simulink model "BulbaBot_ControlLoop"  (R2021b)
settings: Solver=FixedStepAuto  StartTime=0.0  StopTime=2  FixedStep=1e-5  RelTol=1e-3
model workspace (MAT data in the model file):
  PWM_sampleTime = 1e-05
  xG = 0.01
  xd = 189
  yG = 0.01
  yd = 130
  zG = 0.01
  zd = -23
undefined symbols (not defined in the file or in its folder): DiscIntNeverNeededParam
libraries: spsMeanLib x3, simulink x3
settings Model: Creator=Alessandro  LastModifiedBy=Alessandro
settings DataIOCC: ReturnWorkspaceOutputs=off

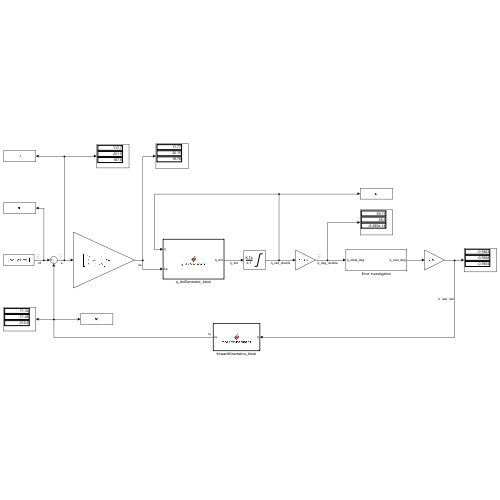
[thumbnail: Simulink's stored preview of the top-level diagram]
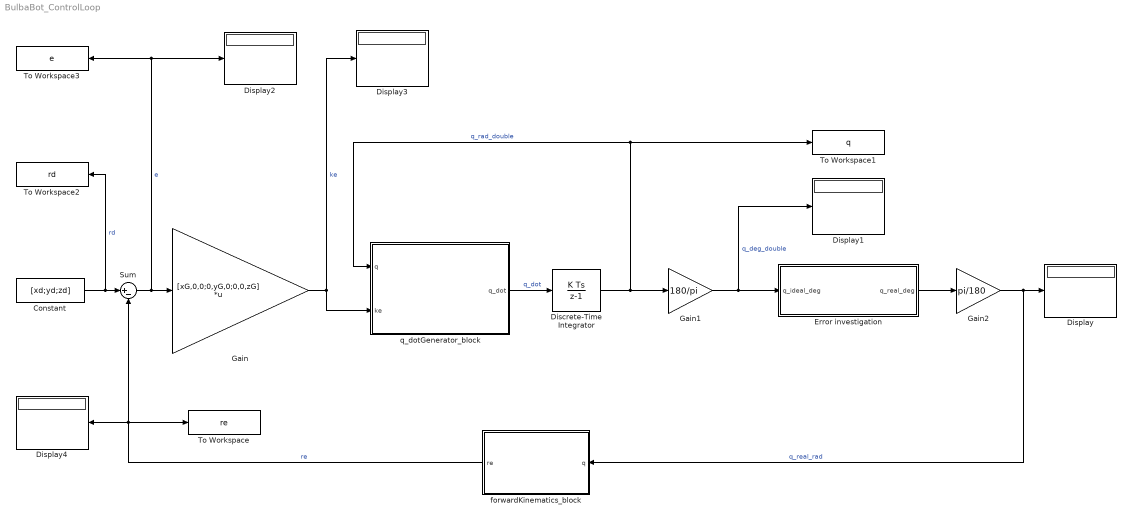
== system BulbaBot_ControlLoop ==
  Constant : Constant  Value=[xd;yd;zd]
  Discrete-Time Integrator : DiscreteIntegrator  InitialCondition=[0,0,0]  SampleTime=-1  LimitOutput=on  UpperSaturationLimit=[pi,pi,pi]  LowerSaturationLimit=[-pi,-pi,-pi]  ICPrevOutput=DiscIntNeverNeededParam  ICPrevScaledInput=DiscIntNeverNeededParam
  Display{,1..4} (5 alike) : Display
  Error investigation : Subsystem
  Gain : Gain  Gain=[xG,0,0;0,yG,0;0,0,zG]  Multiplication=Matrix(K*u)
  Gain1 : Gain  Gain=180/pi
  Gain2 : Gain  Gain=pi/180
  Sum : Sum  Inputs=|+-
  To Workspace : ToWorkspace  VariableName=re  SaveFormat=Timeseries  SampleTime=-1
  To Workspace1 : ToWorkspace  VariableName=q  SaveFormat=Timeseries  SampleTime=-1
  To Workspace2 : ToWorkspace  VariableName=rd  SaveFormat=Timeseries  SampleTime=-1
  To Workspace3 : ToWorkspace  VariableName=e  SaveFormat=Timeseries  SampleTime=-1
  forwardKinematics_block : MATLAB Function  TreatAsAtomicUnit=on
  q_dotGenerator_block : MATLAB Function  TreatAsAtomicUnit=on
  wires:
  Constant/1 -> To Workspace2/1, Sum/1  "rd"
  forwardKinematics_block/1(re) -> To Workspace/1, Display4/1, Sum/2  "re"
  Gain/1 -> q_dotGenerator_block/2(ke), Display3/1  "ke"
  Gain1/1 -> Error investigation/1(q_ideal_deg), Display1/1  "q_deg_double"
  Discrete-Time Integrator/1 -> To Workspace1/1, q_dotGenerator_block/1(q), Gain1/1  "q_rad_double"
  Sum/1 -> To Workspace3/1, Display2/1, Gain/1  "e"
  q_dotGenerator_block/1(q_dot) -> Discrete-Time Integrator/1  "q_dot"
  Gain2/1 -> forwardKinematics_block/1(q), Display/1  "q_real_rad"
  Error investigation/1(q_real_deg) -> Gain2/1

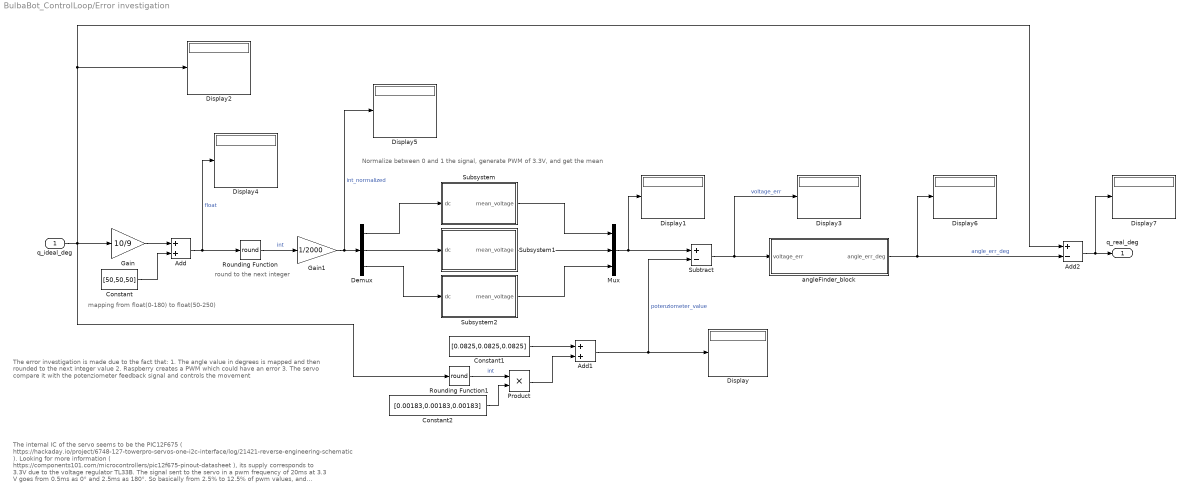
== system BulbaBot_ControlLoop/Error investigation ==
  note: Normalize between 0 and 1 the signal, generate PWM of 3.3V, and get the mean
  note: The internal IC of the servo seems to be the PIC12F675 ( https://hackaday.io/project/6748-127-towerpro-servos-one-i2c-interface/log/21421-reverse-engineering-schematic ).
      |
      | Looking for more information ( https://components101.com/microcontrollers/pic12f675-pinout-datasheet ), its supply corresponds to 3.3V due to the voltage regulator TL33B.
      |
      | The signal sent to the servo in a pwm frequency of 20ms at 3.3 V goes from 0.5ms as 0° and 2.5ms as 180°.
      | So basically from 2.5% to 12.5% of pwm values, and [0.0825,0.4125] V.
  note: round to the next integer
  note: mapping from float(0-180) to float(50-250)
  note: The error investigation is made due to the fact that:
      |
      | 1. The angle value in degrees is mapped and then rounded to the next integer value
      | 2. Raspberry creates a PWM which could have an error
      | 3. The servo compare it with the potenziometer feedback signal and controls the movement
  q_ideal_deg : Inport
  Add : Sum
  Add1 : Sum
  Add2 : Sum  Inputs=+-
  Constant : Constant  Value=[50,50,50]
  Constant1 : Constant  Value=[0.0825,0.0825,0.0825]
  Constant2 : Constant  Value=[0.00183,0.00183,0.00183]
  Demux : Demux  Outputs=3
  Display{,1..7} (8 alike) : Display
  Gain : Gain  Gain=10/9
  Gain1 : Gain  Gain=1/2000
  Mux : Mux  Inputs=3
  Product : Product
  Rounding Function : Rounding  Operator=round
  Rounding Function1 : Rounding  Operator=round
  Subsystem : Subsystem
  Subsystem1 : Subsystem
  Subsystem2 : Subsystem
  Subtract : Sum  Inputs=+-
  angleFinder_block : MATLAB Function  TreatAsAtomicUnit=on
  q_real_deg : Outport
  wires:
  q_ideal_deg/1 -> Add2/1, Display2/1, Rounding Function1/1, Gain/1
  Gain/1 -> Add/1
  Add/1 -> Rounding Function/1, Display4/1  "float"
  Constant/1 -> Add/2
  Rounding Function/1 -> Gain1/1  "int"
  Subtract/1 -> Display3/1, angleFinder_block/1(voltage_err)  "voltage_err"
  angleFinder_block/1(angle_err_deg) -> Add2/2, Display6/1  "angle_err_deg"
  Mux/1 -> Subtract/1, Display1/1
  Gain1/1 -> Display5/1, Demux/1  "int_normalized"
  Demux/1 -> Subsystem/1(dc)
  Demux/2 -> Subsystem1/1(dc)
  Demux/3 -> Subsystem2/1(dc)
  Subsystem/1(mean_voltage) -> Mux/1
  Subsystem1/1(mean_voltage) -> Mux/2
  Subsystem2/1(mean_voltage) -> Mux/3
  Add1/1 -> Subtract/2, Display/1  "potenziometer_value"
  Constant1/1 -> Add1/1
  Product/1 -> Add1/2
  Rounding Function1/1 -> Product/1  "int"
  Constant2/1 -> Product/2
  Add2/1 -> Display7/1, q_real_deg/1

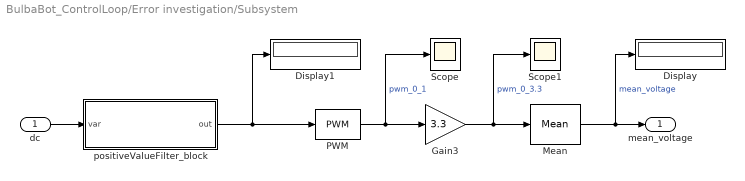
== system BulbaBot_ControlLoop/Error investigation/Subsystem ==
  dc : Inport
  Display : Display
  Display1 : Display
  Gain3 : Gain  Gain=3.3
  Mean : spsMeanLib/Mean  Freq=50  Vinit=0  Ts=0
  PWM : simulink/Discontinuities/PWM  DisableCoverage=on  Period=0.02  DisallowZeroDutyCycle=off  RunAtFixedTimeIntervals=on  SampleTime=PWM_sampleTime
  Scope : Scope
  Scope1 : Scope
  positiveValueFilter_block : MATLAB Function  TreatAsAtomicUnit=on
  mean_voltage : Outport
  wires:
  Gain3/1 -> Scope1/1, Mean/1  "pwm_0_3.3"
  PWM/1 -> Gain3/1, Scope/1  "pwm_0_1"
  Mean/1 -> Display/1, mean_voltage/1  "mean_voltage"
  dc/1 -> positiveValueFilter_block/1(var)
  positiveValueFilter_block/1(out) -> Display1/1, PWM/1

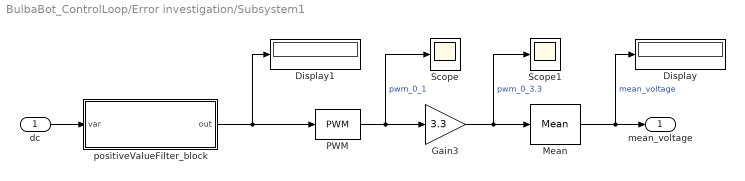
== system BulbaBot_ControlLoop/Error investigation/Subsystem1 ==
  dc : Inport
  Display : Display
  Display1 : Display
  Gain3 : Gain  Gain=3.3
  Mean : spsMeanLib/Mean  Freq=50  Vinit=0  Ts=0
  PWM : simulink/Discontinuities/PWM  DisableCoverage=on  Period=0.02  DisallowZeroDutyCycle=off  RunAtFixedTimeIntervals=on  SampleTime=PWM_sampleTime
  Scope : Scope
  Scope1 : Scope
  positiveValueFilter_block : MATLAB Function  TreatAsAtomicUnit=on
  mean_voltage : Outport
  wires:
  Gain3/1 -> Scope1/1, Mean/1  "pwm_0_3.3"
  PWM/1 -> Gain3/1, Scope/1  "pwm_0_1"
  Mean/1 -> Display/1, mean_voltage/1  "mean_voltage"
  dc/1 -> positiveValueFilter_block/1(var)
  positiveValueFilter_block/1(out) -> Display1/1, PWM/1

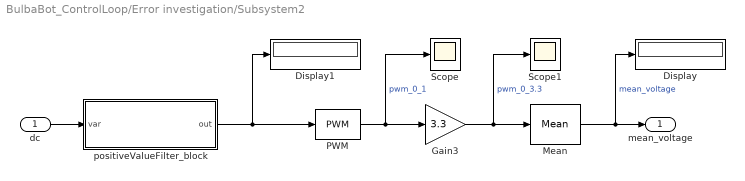
== system BulbaBot_ControlLoop/Error investigation/Subsystem2 ==
  dc : Inport
  Display : Display
  Display1 : Display
  Gain3 : Gain  Gain=3.3
  Mean : spsMeanLib/Mean  Freq=50  Vinit=0  Ts=0
  PWM : simulink/Discontinuities/PWM  DisableCoverage=on  Period=0.02  DisallowZeroDutyCycle=off  RunAtFixedTimeIntervals=on  SampleTime=PWM_sampleTime
  Scope : Scope
  Scope1 : Scope
  positiveValueFilter_block : MATLAB Function  TreatAsAtomicUnit=on
  mean_voltage : Outport
  wires:
  Gain3/1 -> Scope1/1, Mean/1  "pwm_0_3.3"
  PWM/1 -> Gain3/1, Scope/1  "pwm_0_1"
  Mean/1 -> Display/1, mean_voltage/1  "mean_voltage"
  dc/1 -> positiveValueFilter_block/1(var)
  positiveValueFilter_block/1(out) -> Display1/1, PWM/1

== matlab function BulbaBot_ControlLoop/Error investigation/Subsystem/positiveValueFilter_block ==
  data: var input; out output
function out = positiveValueFilter(var)
% DEFINITION:    Function used to delete values lower than 0

% INPUT:         var = in value

% OUTPUT:        out = only positive value or 0

    if var < 0
        out = 0;
    else
        out = var;
    end
end

== matlab function BulbaBot_ControlLoop/q_dotGenerator_block ==
  data: q input; q_dot output; ke input
function q_dot = q_dotGenerator(q,ke)
% DEFINITION:    The evaluation of the Jacobian permits to get the value of
%                q_dot, which after has been integrated begin the needed q

% INPUT:         q = quantized rounded expected angle
%                ke = results of the multiplication of the error with the gain correction

% OUTPUT:        q_dot = angular velocity in rads/s of the joints

%% Jacobian computation
%   Computation made in J_T_evaluation
    q1 = q(1);
    q2 = q(2);
    q3 = q(3);

    J1 = [- (101*sin(q1))/2 - 160*sin(q3)*((4967757600021511*cos(q1)*cos(q2))/81129638414606681695789005144064 - sin(q1)*sin(q2)) - (710389336803076073*cos(q1)*sin(q2))/162259276829213363391578010288128 - (143*cos(q2)*sin(q1))/2 - 160*cos(q3)*((4967757600021511*cos(q1)*sin(q2))/81129638414606681695789005144064 + cos(q2)*sin(q1)), - 160*sin(q3)*(cos(q1)*cos(q2) - (4967757600021511*sin(q1)*sin(q2))/81129638414606681695789005144064) - (143*cos(q1)*sin(q2))/2 - (710389336803076073*cos(q2)*sin(q1))/162259276829213363391578010288128 - 160*cos(q3)*(cos(q1)*sin(q2) + (4967757600021511*cos(q2)*sin(q1))/81129638414606681695789005144064), - 160*sin(q3)*(cos(q1)*cos(q2) - (4967757600021511*sin(q1)*sin(q2))/81129638414606681695789005144064) - 160*cos(q3)*(cos(q1)*sin(q2) + (4967757600021511*cos(q2)*sin(q1))/81129638414606681695789005144064)];
    J2 = [  (101*cos(q1))/2 - 160*sin(q3)*(cos(q1)*sin(q2) + (4967757600021511*cos(q2)*sin(q1))/81129638414606681695789005144064) + (143*cos(q1)*cos(q2))/2 - (710389336803076073*sin(q1)*sin(q2))/162259276829213363391578010288128 + 160*cos(q3)*(cos(q1)*cos(q2) - (4967757600021511*sin(q1)*sin(q2))/81129638414606681695789005144064),   (710389336803076073*cos(q1)*cos(q2))/162259276829213363391578010288128 - 160*sin(q3)*((4967757600021511*cos(q1)*sin(q2))/81129638414606681695789005144064 + cos(q2)*sin(q1)) - (143*sin(q1)*sin(q2))/2 + 160*cos(q3)*((4967757600021511*cos(q1)*cos(q2))/81129638414606681695789005144064 - sin(q1)*sin(q2)),   160*cos(q3)*((4967757600021511*cos(q1)*cos(q2))/81129638414606681695789005144064 - sin(q1)*sin(q2)) - 160*sin(q3)*((4967757600021511*cos(q1)*sin(q2))/81129638414606681695789005144064 + cos(q2)*sin(q1))];
    J3 = [                                                                                                                                                                                                                                                                                                                               0,                                                                                                                                                                                                                                                    (143*cos(q2))/2 + 160*cos(q2)*cos(q3) - 160*sin(q2)*sin(q3),                                                                                                                                                                   160*cos(q2)*cos(q3) - 160*sin(q2)*sin(q3)];
 
    J = [J1;J2;J3];

%% Result evaluation
%     q_dot = J'*ke*e
    q1_dot = J(1,1)*ke(1)+J(2,1)*ke(2)+J(3,1)*ke(3);
    q2_dot = J(1,2)*ke(1)+J(2,2)*ke(2)+J(3,2)*ke(3);
    q3_dot = J(1,3)*ke(1)+J(2,3)*ke(2)+J(3,3)*ke(3);
    q_dot = [q1_dot,q2_dot,q3_dot];
end

== matlab function BulbaBot_ControlLoop/Error investigation/angleFinder_block ==
  data: voltage_err input; angle_err_deg output
function angle_err_deg = angleFinder(voltage_err)
% DEFINITION:    Function used to map the voltage error from the
%                comparator into a real angle error that can be used to correct the
%                overral error

% INPUT:         voltage_err = output of the comparator 

% OUTPUT:        angle_err_deg = real angle error in degrees

    %map voltage error from 0/3.3 V to 0/20 ms 
    pwm_dc_err = voltage_err.*0.02./3.3;

    %map error from 0.5/2.5 ms to 0/180
    angle_err_deg = zeros(1,length(pwm_dc_err));
    for i = 1:length(pwm_dc_err)
        if abs(pwm_dc_err(i))<0.0005 %mean that the error is less than 0°
            angle_err_deg(i) = 0;
        else
            if pwm_dc_err(i) >= 0
                angle_err_deg(i) = 90000*pwm_dc_err(i)-45;
            else
                angle_err_deg(i) = pwm_dc_err(i)*90000+45;
            end
        end
    end
end

== matlab function BulbaBot_ControlLoop/forwardKinematics_block ==
  data: re output; q input
function re = forwardKinematics(q)
% DEFINITION:    after had evaluated the error of the servo through caused from
%                its internal quantization of rounded angle forward kinematics is applied
%                in order to get the expected real value of the position and use it into
%                simulink to get the error

% INPUT:         q = quantized rounded expected angle

% OUTPUT:        re = expected real position of the end effector

%% Generation of the T matrix with the aim of DH convention formula
%     With the following method the T03 matrix is evaluated at each iteration
%     T = eye(4);
%     for i = 1:3
%         T = T * [cos(q(i)),-sin(q(i))*cos(alpha(i)),sin(q(i))*sin(alpha(i)),a(i)*cos(q(i));
%                  sin(q(i)),cos(q(i))*cos(alpha(i)),-cos(q(i))*sin(alpha(i)),a(i)*sin(q(i));
%                  0,sin(alpha(i)),cos(alpha(i)),d(i);
%                  0,0,0,1];
%     end

%     To simplify computation complexity, I evaluated T03 in J_T_evaluation
    q1 = q(1);
    q2 = q(2);
    q3 = q(3);

    T1 = [cos(q3)*(cos(q1)*cos(q2) - (4967757600021511*sin(q1)*sin(q2))/81129638414606681695789005144064) - sin(q3)*(cos(q1)*sin(q2) + (4967757600021511*cos(q2)*sin(q1))/81129638414606681695789005144064), - sin(q3)*(cos(q1)*cos(q2) - (4967757600021511*sin(q1)*sin(q2))/81129638414606681695789005144064) - cos(q3)*(cos(q1)*sin(q2) + (4967757600021511*cos(q2)*sin(q1))/81129638414606681695789005144064),                                           sin(q1), (101*cos(q1))/2 - 160*sin(q3)*(cos(q1)*sin(q2) + (4967757600021511*cos(q2)*sin(q1))/81129638414606681695789005144064) + (143*cos(q1)*cos(q2))/2 - (710389336803076073*sin(q1)*sin(q2))/162259276829213363391578010288128 + 160*cos(q3)*(cos(q1)*cos(q2) - (4967757600021511*sin(q1)*sin(q2))/81129638414606681695789005144064)];
    T2 = [sin(q3)*((4967757600021511*cos(q1)*cos(q2))/81129638414606681695789005144064 - sin(q1)*sin(q2)) + cos(q3)*((4967757600021511*cos(q1)*sin(q2))/81129638414606681695789005144064 + cos(q2)*sin(q1)),   cos(q3)*((4967757600021511*cos(q1)*cos(q2))/81129638414606681695789005144064 - sin(q1)*sin(q2)) - sin(q3)*((4967757600021511*cos(q1)*sin(q2))/81129638414606681695789005144064 + cos(q2)*sin(q1)),                                          -cos(q1), (101*sin(q1))/2 + 160*sin(q3)*((4967757600021511*cos(q1)*cos(q2))/81129638414606681695789005144064 - sin(q1)*sin(q2)) + (710389336803076073*cos(q1)*sin(q2))/162259276829213363391578010288128 + (143*cos(q2)*sin(q1))/2 + 160*cos(q3)*((4967757600021511*cos(q1)*sin(q2))/81129638414606681695789005144064 + cos(q2)*sin(q1))];
    T3 = [                                                                                                                                                                cos(q2)*sin(q3) + cos(q3)*sin(q2),                                                                                                                                                                   cos(q2)*cos(q3) - sin(q2)*sin(q3), 4967757600021511/81129638414606681695789005144064,                                                                                                                                                                                                                                                                    (143*sin(q2))/2 + 160*cos(q2)*sin(q3) + 160*cos(q3)*sin(q2)];
    T4 = [                                                                                                                                                                                                0,                                                                                                                                                                                                   0,                                                 0,                                                                                                                                                                                                                                                                                                                              1];
 
    T = [T1;T2;T3;T4];
    
    xe = T(1,4);
    ye = T(2,4);
    ze = T(3,4);

    re = [xe;ye;ze];
end

== matlab function BulbaBot_ControlLoop/Error investigation/Subsystem1/positiveValueFilter_block ==
  data: var input; out output
function out = positiveValueFilter(var)
% DEFINITION:    Function used to delete values lower than 0

% INPUT:         var = in value

% OUTPUT:        out = only positive value or 0

    if var < 0
        out = 0;
    else
        out = var;
    end
end

== matlab function BulbaBot_ControlLoop/Error investigation/Subsystem2/positiveValueFilter_block ==
  data: var input; out output
function out = positiveValueFilter(var)
% DEFINITION:    Function used to delete values lower than 0

% INPUT:         var = in value

% OUTPUT:        out = only positive value or 0

    if var < 0
        out = 0;
    else
        out = var;
    end
end
